simulink model "FocHFIGenerator"  (R2024a)
settings: Solver=FixedStepDiscrete  StartTime=0.0  StopTime=1  FixedStep=0.00005  RelTol=1e-3
values from neighbouring files (symbols this model uses):
  Max_Current = 10    [FocHFIGenerator.mat]    (also in NLFO_CodeGenerator.mat)
  Pole = 10    [FocHFIGenerator.mat]    (also in NLFO_CodeGenerator.mat = 7)
  UdInjectVal = 2.5    [FocHFIGenerator.mat]
undefined symbols (not defined in the file or in its folder): DiscIntNeverNeededParam
libraries: slpidlib x4
settings Model: Creator=张先生  LastModifiedBy=张先生
settings OptimizationCC: DefaultParameterBehavior=Inlined  UseDivisionForNetSlopeComputation=on  GainParamInheritBuiltInType=on  UseFloatMulNetSlope=on  InlineInvariantSignals=on  PassReuseOutputArgsAs=Individual arguments  ZeroExternalMemoryAtStartup=off  ZeroInternalMemoryAtStartup=off  NoFixptDivByZeroProtection=on  EfficientFloat2IntCast=on  LifeSpan=1  OptimizeBlockOrder=speed  DifferentSizesBufferReuse=on  EfficientTunableParamExpr=on
settings DebuggingCC: ParameterTunabilityLossMsg=error
settings HardwareCC: ProdBitPerPointer=32  ProdBitPerSizeT=32  ProdBitPerPtrDiffT=32  ProdLargestAtomicInteger=Long  ProdLargestAtomicFloat=Double  ProdWordSize=32  ProdLongLongMode=on  ProdHWDeviceType=ARM Compatible->ARM Cortex-M
settings SFSimCC: MATLABDynamicMemAlloc=off
settings RTWCC: Description=Embedded Coder  SystemTargetFile=ert.tlc  TemplateMakefile=ert_default_tmf  GenerateReport=on  LaunchReport=on
settings CodeAppCC: ForceParamTrailComments=on  IgnoreCustomStorageClasses=off  OperatorAnnotations=on  SimulinkDataObjDesc=on  SFDataObjDesc=on  CustomSymbolStrGlobalVar=rt$N$M  CustomSymbolStrType=$N$M  CustomSymbolStrFcn=$N$M$F  CustomSymbolStrMacro=$N$M  InsertBlockDesc=on
settings ERTTargetCC: TargetLangStandard=C99 (ISO)  CodeReplacementLibrary=ARM Cortex-M  GenerateSampleERTMain=on  IncludeMdlTerminateFcn=off  CombineSignalStateStructs=on  SupportComplex=off  SupportContinuousTime=on  InlinedParameterPlacement=NonHierarchical  ERTCustomFileTemplate=example_file_process.tlc  ERTFilePackagingFormat=CompactWithDataFile

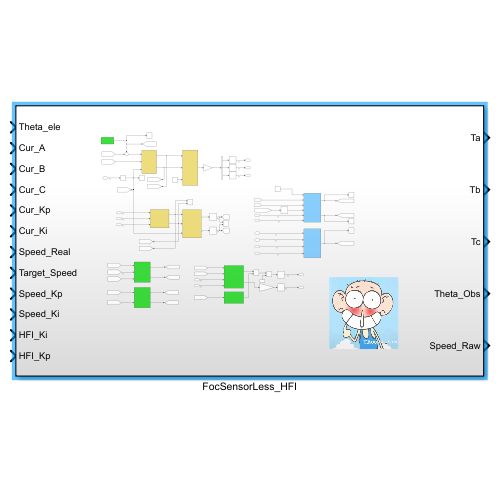
[thumbnail: Simulink's stored preview of the top-level diagram]
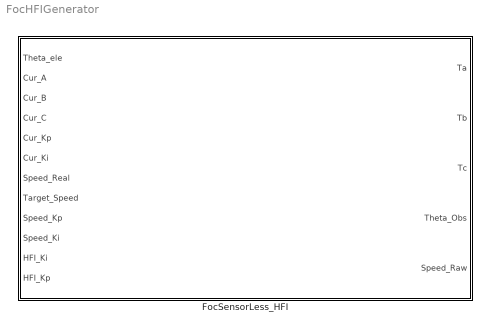
== system FocHFIGenerator ==
  FocSensorLess_HFI : Subsystem

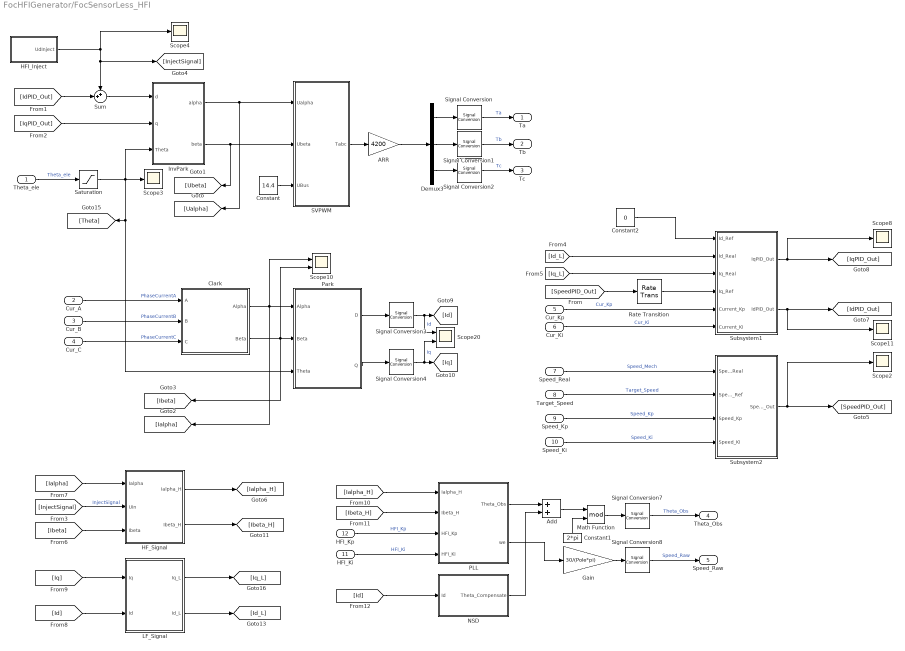
== system FocHFIGenerator/FocSensorLess_HFI ==
  Theta_ele : Inport
  Cur_A : Inport  Port=2
  Cur_B : Inport  Port=3
  Cur_C : Inport  Port=4
  Cur_Kp : Inport  Port=5
  Cur_Ki : Inport  Port=6
  Speed_Real : Inport  Port=7
  Target_Speed : Inport  Port=8
  Speed_Kp : Inport  Port=9
  Speed_Ki : Inport  Port=10
  HFI_Ki : Inport  Port=11
  HFI_Kp : Inport  Port=12
  ARR : Gain  Gain=4200
  Add : Sum
  Clark : Subsystem  TreatAsAtomicUnit=on
      settings: RTWSystemCode=Inline  RTWFcnNameOpts=Use subsystem name
      mask Display:
      | port_label('input',1,'a','texmode','on');
      | port_label('input',2,'b','texmode','on');
      | port_label('input',3,'c','texmode','on');
      | 
      | port_label('output',1,'\alpha','texmode','on');
      | port_label('output',2,'\beta','texmode','on');
      | 
      | fprintf('Clark');
  Constant : Constant  Value=14.4  OutDataTypeStr=single
  Constant1 : Constant  Value=2*pi  OutDataTypeStr=single
  Constant2 : Constant  Value=0  OutDataTypeStr=single
  Demux3 : Demux  Outputs=3
  Gain : Gain  Gain=30/(Pole*pi)
  HFI_Inject : Subsystem
  HF_Signal : Subsystem
  InvPark : Subsystem  TreatAsAtomicUnit=on
      settings: RTWFcnNameOpts=Use subsystem name
      mask Display:
      | port_label('input',1,'d','texmode','on');
      | port_label('input',2,'q','texmode','on');
      | port_label('input',3,'\theta','texmode','on');
      | 
      | port_label('output',1,'\alpha','texmode','on');
      | port_label('output',2,'\beta','texmode','on');
      | 
      | fprintf('Inverse\nPark')
  LF_Signal : Subsystem
  Math Function : Math  Operator=mod
  NSD : Subsystem
  PLL : Subsystem
  Park : Subsystem  TreatAsAtomicUnit=on
      settings: RTWFcnNameOpts=Use subsystem name
      mask Display:
      | port_label('input',1,'\alpha','texmode','on');
      | port_label('input',2, '\beta','texmode','on');
      | port_label('input',3, '\theta','texmode','on');
      | 
      | port_label('output',1,'d','texmode','on');
      | port_label('output',2,'q','texmode','on');
      | fprintf('Park');
  Rate Transition : RateTransition
  SVPWM : Subsystem  TreatAsAtomicUnit=on
  Saturation : Saturate  UpperLimit=2*pi-0.001  LowerLimit=-2*pi + 0.001
  Scope10 : Scope  NumInputPorts=2
  Scope{2..4,8,11} (5 alike) : Scope
  Scope20 : Scope  NumInputPorts=2
  Signal Conversion{,1..4,7..8} (7 alike) : SignalConversion  OverrideOpt=off
  Subsystem1 : Subsystem
  Subsystem2 : Subsystem
  Sum : Sum  Inputs=++|
  Ta : Outport
  Tb : Outport  Port=2
  Tc : Outport  Port=3
  Theta_Obs : Outport  Port=4
  Speed_Raw : Outport  Port=5
  wires:
  [Id_L] -> Subsystem1/2(Id_Real)
  InvPark/1(alpha) -> SVPWM/1(Ualpha), [Ualpha]
  InvPark/2(beta) -> SVPWM/2(Ubeta), [Ubeta]
  Saturation/1 -> [Theta], Park/3(Theta), Scope3/1, InvPark/3(Theta)
  Cur_Kp/1 -> Subsystem1/5(Current_Kp)  "Cur_Kp"
  SVPWM/1(Tabc) -> ARR/1
  Subsystem1/1(IqPID_Out) -> Scope8/1, [IqPID_Out]
  Theta_ele/1 -> Saturation/1  "Theta_ele"
  ARR/1 -> Demux3/1
  Cur_C/1 -> Clark/3(C)  "PhaseCurrentC"
  Park/1(D) -> Signal Conversion3/1
  Signal Conversion4/1 -> Scope20/2, [Iq]  "Iq"
  Cur_B/1 -> Clark/2(B)  "PhaseCurrentB"
  Signal Conversion2/1 -> Tc/1  "Tc"
  Signal Conversion3/1 -> Scope20/1, [Id]  "Id"
  Signal Conversion/1 -> Ta/1  "Ta"
  Cur_A/1 -> Clark/1(A)  "PhaseCurrentA"
  Demux3/2 -> Signal Conversion1/1
  Demux3/1 -> Signal Conversion/1
  Park/2(Q) -> Signal Conversion4/1
  [Iq_L] -> Subsystem1/3(Iq_Real)
  Demux3/3 -> Signal Conversion2/1
  Subsystem1/2(IdPID_Out) -> Scope11/1, [IdPID_Out]
  Signal Conversion1/1 -> Tb/1  "Tb"
  Constant/1 -> SVPWM/3(UBus)
  Cur_Ki/1 -> Subsystem1/6(Current_Ki)  "Cur_Ki"
  Subsystem2/1(SpeedPID_Out) -> Scope2/1, [SpeedPID_Out]
  [SpeedPID_Out] -> Rate Transition/1
  Speed_Real/1 -> Subsystem2/1(Speed_Real)  "Speed_Mech"
  Target_Speed/1 -> Subsystem2/2(Speed_Ref)  "Target_Speed"
  Speed_Kp/1 -> Subsystem2/3(Speed_Kp)  "Speed_Kp"
  Speed_Ki/1 -> Subsystem2/4(Speed_Ki)  "Speed_Ki"
  Rate Transition/1 -> Subsystem1/4(Iq_Ref)
  Clark/2(Beta) -> [Ibeta], Park/2(Beta), Scope10/2
  Clark/1(Alpha) -> [Ialpha], Park/1(Alpha), Scope10/1
  Sum/1 -> InvPark/1(d)
  HFI_Inject/1(UdInject) -> Scope4/1, Sum/1, [InjectSignal]
  HFI_Ki/1 -> PLL/4(HFI_Ki)  "HFI_Ki"
  HFI_Kp/1 -> PLL/3(HFI_Kp)  "HFI_Kp"
  [Ibeta_H] -> PLL/2(Ibeta_H)
  [Ialpha_H] -> PLL/1(Ialpha_H)
  PLL/1(Theta_Obs) -> Add/1
  NSD/1(Theta_Compensate) -> Add/2
  Constant1/1 -> Math Function/2
  Add/1 -> Math Function/1
  Math Function/1 -> Signal Conversion7/1
  PLL/2(we) -> Gain/1
  Signal Conversion7/1 -> Theta_Obs/1  "Theta_Obs"
  Signal Conversion8/1 -> Speed_Raw/1  "Speed_Raw"
  [Ibeta] -> HF_Signal/3(Ibeta)
  [Ialpha] -> HF_Signal/1(Ialpha)
  [InjectSignal] -> HF_Signal/2(Uin)  "InjectSignal"
  HF_Signal/2(Ibeta_H) -> [Ibeta_H]
  HF_Signal/1(Ialpha_H) -> [Ialpha_H]
  [Iq] -> LF_Signal/1(Iq)
  [Id] -> LF_Signal/2(Id)
  LF_Signal/1(Iq_L) -> [Iq_L]
  LF_Signal/2(Id_L) -> [Id_L]
  [Id] -> NSD/1(Id)
  Gain/1 -> Signal Conversion8/1
  Constant2/1 -> Subsystem1/1(Id_Ref)
  [IdPID_Out] -> Sum/2
  [IqPID_Out] -> InvPark/2(q)

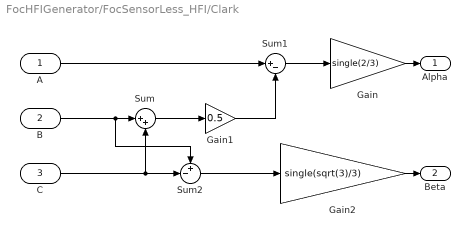
== system FocHFIGenerator/FocSensorLess_HFI/Clark ==
  A : Inport  OutDataTypeStr=single
  B : Inport  Port=2  OutDataTypeStr=single
  C : Inport  Port=3  OutDataTypeStr=single
  Gain : Gain  Gain=single(2/3)  OutDataTypeStr=single
  Gain1 : Gain  Gain=0.5  OutDataTypeStr=single
  Gain2 : Gain  Gain=single(sqrt(3)/3)  OutDataTypeStr=single
  Sum : Sum  Inputs=|++  OutDataTypeStr=single
  Sum1 : Sum  Inputs=|+-  OutDataTypeStr=single
  Sum2 : Sum  Inputs=+-|  OutDataTypeStr=single
  Alpha : Outport  OutDataTypeStr=single
  Beta : Outport  Port=2  OutDataTypeStr=single
  wires:
  Sum/1 -> Gain1/1
  Gain2/1 -> Beta/1
  B/1 -> Sum2/1, Sum/1
  Gain1/1 -> Sum1/2
  Gain/1 -> Alpha/1
  Sum2/1 -> Gain2/1
  C/1 -> Sum2/2, Sum/2
  A/1 -> Sum1/1
  Sum1/1 -> Gain/1

== system FocHFIGenerator/FocSensorLess_HFI/HFI_Inject ==
  note: 前0.2S进行极性辨识
  Scope : Scope
  Scope1 : Scope  NumInputPorts=2
  Subsystem : Subsystem
  Subsystem4 : Subsystem
  Sum1 : Sum  Inputs=++|
  UdInject : Outport
  wires:
  Subsystem/1(Ud_Inject) -> Scope1/2, Sum1/2
  Subsystem4/1(NDS_Signal) -> Scope1/1, Sum1/1
  Sum1/1 -> Scope/1, UdInject/1

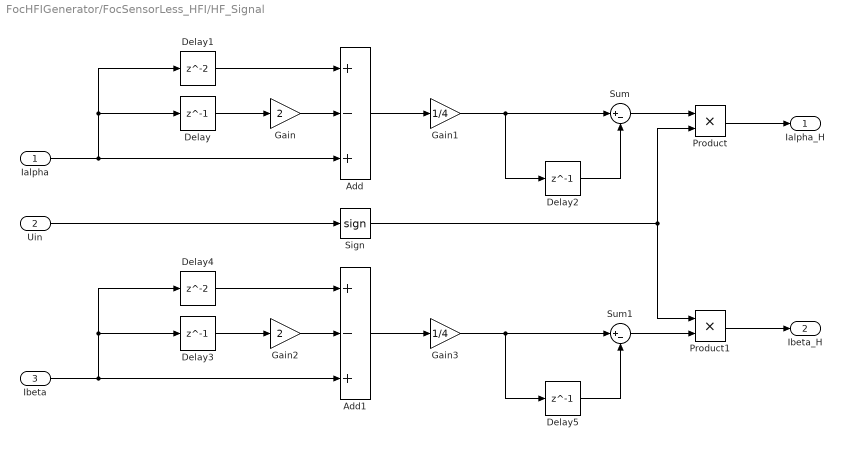
== system FocHFIGenerator/FocSensorLess_HFI/HF_Signal ==
  Ialpha : Inport
  Uin : Inport  Port=2
  Ibeta : Inport  Port=3
  Add : Sum  Inputs=+-+
  Add1 : Sum  Inputs=+-+
  Delay{,2..3,5} (4 alike) : Delay  DelayLength=1
  Delay1 : Delay
  Delay4 : Delay
  Gain : Gain  Gain=2
  Gain1 : Gain  Gain=1/4
  Gain2 : Gain  Gain=2
  Gain3 : Gain  Gain=1/4
  Product : Product
  Product1 : Product
  Sign : Signum
  Sum : Sum  Inputs=|+-
  Sum1 : Sum  Inputs=|+-
  Ialpha_H : Outport
  Ibeta_H : Outport  Port=2
  wires:
  Delay/1 -> Gain/1
  Delay1/1 -> Add/1
  Gain/1 -> Add/2
  Ialpha/1 -> Add/3, Delay1/1, Delay/1
  Add/1 -> Gain1/1
  Gain1/1 -> Delay2/1, Sum/1
  Delay2/1 -> Sum/2
  Sum/1 -> Product/1
  Product/1 -> Ialpha_H/1
  Uin/1 -> Sign/1
  Sign/1 -> Product1/1, Product/2
  Product1/1 -> Ibeta_H/1
  Add1/1 -> Gain3/1
  Delay5/1 -> Sum1/2
  Gain3/1 -> Delay5/1, Sum1/1
  Delay4/1 -> Add1/1
  Gain2/1 -> Add1/2
  Ibeta/1 -> Add1/3, Delay4/1, Delay3/1
  Delay3/1 -> Gain2/1
  Sum1/1 -> Product1/2

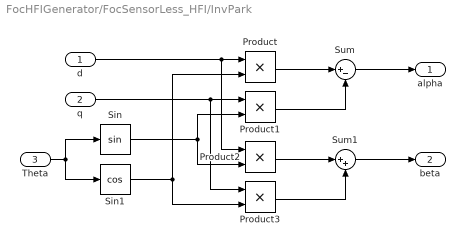
== system FocHFIGenerator/FocSensorLess_HFI/InvPark ==
  d : Inport  OutDataTypeStr=single
  q : Inport  Port=2  OutDataTypeStr=single
  Theta : Inport  Port=3  OutDataTypeStr=single
  Product{,1..3} (4 alike) : Product  OutDataTypeStr=single
  Sin : Trigonometry  ApproximationMethod=Lookup  TableDataTypeStr=single
  Sin1 : Trigonometry  Operator=cos  ApproximationMethod=Lookup  TableDataTypeStr=single
  Sum : Sum  Inputs=|+-  OutDataTypeStr=single
  Sum1 : Sum  Inputs=|++  OutDataTypeStr=single
  alpha : Outport  OutDataTypeStr=single
  beta : Outport  Port=2  OutDataTypeStr=single
  wires:
  Sum/1 -> alpha/1
  Theta/1 -> Sin1/1, Sin/1
  d/1 -> Product2/1, Product/1
  Sin1/1 -> Product/2, Product3/2
  q/1 -> Product3/1, Product1/1
  Sin/1 -> Product1/2, Product2/2
  Product/1 -> Sum/1
  Product1/1 -> Sum/2
  Product2/1 -> Sum1/1
  Product3/1 -> Sum1/2
  Sum1/1 -> beta/1

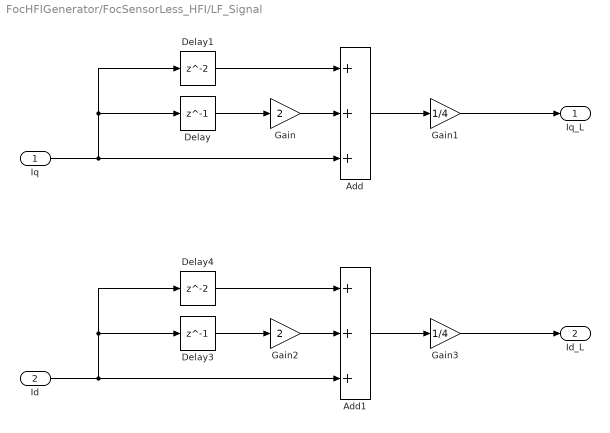
== system FocHFIGenerator/FocSensorLess_HFI/LF_Signal ==
  Iq : Inport
  Id : Inport  Port=2
  Add : Sum  Inputs=+++
  Add1 : Sum  Inputs=+++
  Delay : Delay  DelayLength=1
  Delay1 : Delay
  Delay3 : Delay  DelayLength=1
  Delay4 : Delay
  Gain : Gain  Gain=2
  Gain1 : Gain  Gain=1/4
  Gain2 : Gain  Gain=2
  Gain3 : Gain  Gain=1/4
  Iq_L : Outport
  Id_L : Outport  Port=2
  wires:
  Delay/1 -> Gain/1
  Delay1/1 -> Add/1
  Gain/1 -> Add/2
  Iq/1 -> Add/3, Delay1/1, Delay/1
  Add/1 -> Gain1/1
  Gain1/1 -> Iq_L/1
  Gain3/1 -> Id_L/1
  Add1/1 -> Gain3/1
  Delay4/1 -> Add1/1
  Gain2/1 -> Add1/2
  Id/1 -> Add1/3, Delay4/1, Delay3/1
  Delay3/1 -> Gain2/1

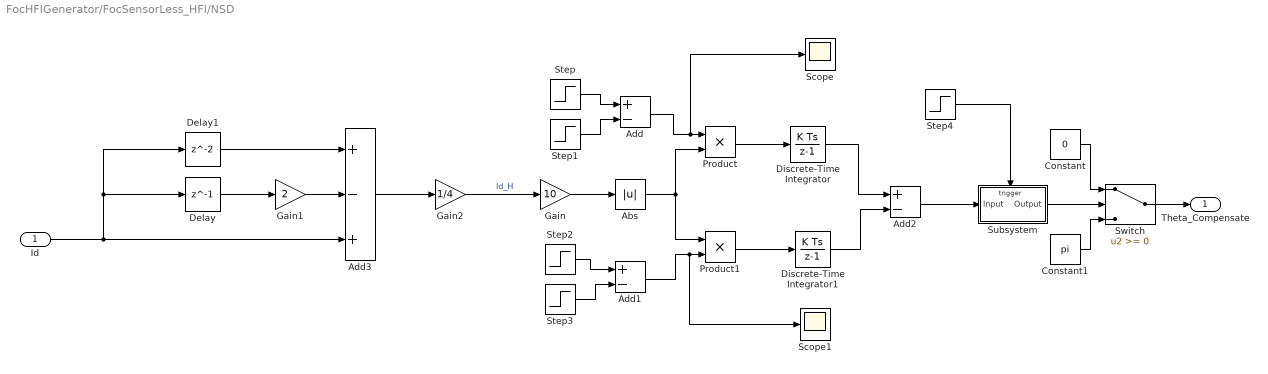
== system FocHFIGenerator/FocSensorLess_HFI/NSD ==
  Id : Inport
  Abs : Abs  OutDataTypeStr=single  SaturateOnIntegerOverflow=off
  Add : Sum  Inputs=+-  OutDataTypeStr=single  AccumDataTypeStr=single
  Add1 : Sum  Inputs=+-  OutDataTypeStr=single  AccumDataTypeStr=single
  Add2 : Sum  Inputs=+-  OutDataTypeStr=single  AccumDataTypeStr=single
  Add3 : Sum  Inputs=+-+
  Constant : Constant  Value=0  OutDataTypeStr=single
  Constant1 : Constant  Value=pi  OutDataTypeStr=single
  Delay : Delay  DelayLength=1
  Delay1 : Delay
  Discrete-Time Integrator : DiscreteIntegrator  SampleTime=-1  OutDataTypeStr=single  ICPrevOutput=DiscIntNeverNeededParam  ICPrevScaledInput=DiscIntNeverNeededParam
  Discrete-Time Integrator1 : DiscreteIntegrator  SampleTime=-1  OutDataTypeStr=single  ICPrevOutput=DiscIntNeverNeededParam  ICPrevScaledInput=DiscIntNeverNeededParam
  Gain : Gain  Gain=10
  Gain1 : Gain  Gain=2
  Gain2 : Gain  Gain=1/4
  Product : Product  OutDataTypeStr=single
  Product1 : Product  OutDataTypeStr=single
  Scope : Scope
  Scope1 : Scope
  Step : Step  Time=0.1  OutDataTypeStr=single  SampleTime=0
  Step1 : Step  Time=0.11  OutDataTypeStr=single  SampleTime=0
  Step2 : Step  Time=0.13  After=-1  OutDataTypeStr=single  SampleTime=0
  Step3 : Step  Time=0.14  After=-1  OutDataTypeStr=single  SampleTime=0
  Step4 : Step  Time=0.15  SampleTime=0
  Subsystem : Subsystem
  Switch : Switch  OutDataTypeStr=single  SaturateOnIntegerOverflow=off  InputSameDT=off
  Theta_Compensate : Outport
  wires:
  Gain/1 -> Abs/1
  Step/1 -> Add/1
  Step1/1 -> Add/2
  Step2/1 -> Add1/1
  Step3/1 -> Add1/2
  Add/1 -> Scope/1, Product/1
  Add1/1 -> Scope1/1, Product1/2
  Abs/1 -> Product1/1, Product/2
  Product/1 -> Discrete-Time Integrator/1
  Product1/1 -> Discrete-Time Integrator1/1
  Discrete-Time Integrator/1 -> Add2/1
  Discrete-Time Integrator1/1 -> Add2/2
  Step4/1 -> Subsystem/Trigger
  Add2/1 -> Subsystem/1(Input)
  Subsystem/1(Output) -> Switch/2
  Constant/1 -> Switch/1
  Constant1/1 -> Switch/3
  Switch/1 -> Theta_Compensate/1
  Id/1 -> Add3/3, Delay1/1, Delay/1
  Gain1/1 -> Add3/2
  Delay1/1 -> Add3/1
  Add3/1 -> Gain2/1
  Delay/1 -> Gain1/1
  Gain2/1 -> Gain/1  "Id_H"

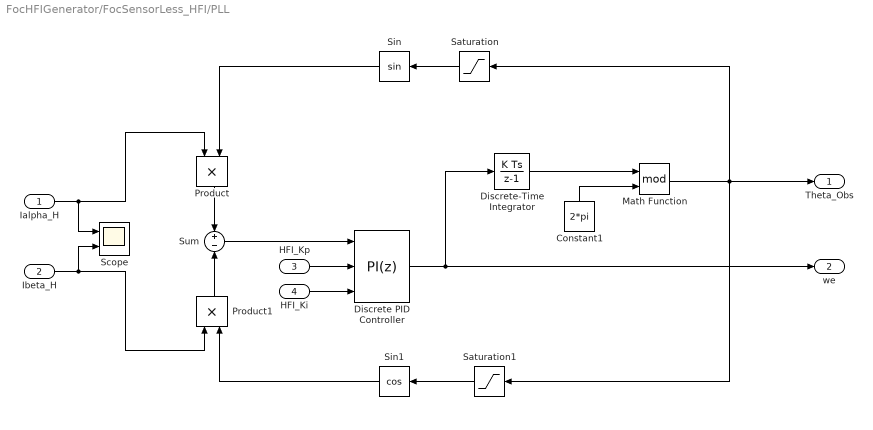
== system FocHFIGenerator/FocSensorLess_HFI/PLL ==
  Ialpha_H : Inport
  Ibeta_H : Inport  Port=2
  HFI_Kp : Inport  Port=3
  HFI_Ki : Inport  Port=4
  Constant1 : Constant  Value=2*pi  OutDataTypeStr=single
  Discrete PID Controller : slpidlib/PID Controller  Controller=PI  Form=Parallel  TimeDomain=Discrete-time  UseExternalTs=off  SampleTime=-1  IntegratorMethod=Forward Euler  FilterMethod=Forward Euler  ControllerParametersSource=external  P=10  I=1000  UseKiTs=off  D=0  UseExternalDerivativeSource=off  N=100  UseFilter=on  TunerSelectOption=Transfer Function Based (PID Tuner App)  InitialConditionSource=internal  InitialConditionForIntegrator=0  InitialConditionForFilter=0  DifferentiatorICPrevScaledInput=0  ExternalReset=none  TrackingMode=off  Kt=1  LimitOutput=off  SatLimitsSource=internal  UpperSaturationLimit=pi*2  LowerSaturationLimit=-pi*2  LinearizeAsGain=on  AntiWindupMode=clamping  Kb=1  LimitIntegrator=off  UpperIntegratorSaturationLimit=inf  LowerIntegratorSaturationLimit=-inf  PGainOutDataTypeStr=single  PProdOutDataTypeStr=single  POutMin=[]  POutMax=[]  IGainOutDataTypeStr=single  IProdOutDataTypeStr=single  IOutMin=[]  IOutMax=[]  DOutMin=[]  DOutMax=[]  NOutMin=[]  NOutMax=[]  SumOutDataTypeStr=single  SumOutMin=[]  SumOutMax=[]  SaturationOutMin=[]  SaturationOutMax=[]  PParamMin=[]  PParamMax=[]  IParamMin=[]  IParamMax=[]  DParamMin=[]  DParamMax=[]  NParamMin=[]  NParamMax=[]  KbParamMin=[]  KbParamMax=[]  KtParamMin=[]  KtParamMax=[]  KbOutMin=[]  KbOutMax=[]  KtOutMin=[]  KtOutMax=[]  IntegratorOutMin=[]  IntegratorOutMax=[]  FilterOutMin=[]  FilterOutMax=[]  SumI1OutMin=[]  SumI1OutMax=[]  SumI2OutMin=[]  SumI2OutMax=[]  SumI3OutMin=[]  SumI3OutMax=[]  SumI4OutMin=[]  SumI4OutMax=[]  SumDOutMin=[]  SumDOutMax=[]  DifferentiatorOutMin=[]  DifferentiatorOutMax=[]  FilterDiffOutCoefMin=[]  FilterDiffOutCoefMax=[]  ReciprocalOutMin=[]  ReciprocalOutMax=[]  SumDenOutMin=[]  SumDenOutMax=[]  SumNumOutMin=[]  SumNumOutMax=[]  DivideOutMin=[]  DivideOutMax=[]  UdiffTsProdOutMin=[]  UdiffTsProdOutMax=[]  NTsProdOutMin=[]  NTsProdOutMax=[]  UintegralTsProdOutMin=[]  UintegralTsProdOutMax=[]  UngainTsProdOutMin=[]  UngainTsProdOutMax=[]  ClampingZeroOutDataTypeStr=Inherit: Inherit via back propagation  ClampingZeroOutMin=[]  ClampingZeroOutMax=[]  FilterDenConstantOutDataTypeStr=Inherit: Inherit via back propagation  FilterDenConstantOutMin=[]  FilterDenConstantOutMax=[]  PCopyOutDataTypeStr=Inherit: Inherit via back propagation  PCopyOutMin=[]  PCopyOutMax=[]  NCopyOutDataTypeStr=Inherit: Inherit via back propagation  NCopyOutMin=[]  NCopyOutMax=[]  IntegratorContinuousStateAttributes=''  IntegratorStateMustResolveToSignalObject=off  IntegratorRTWStateStorageClass=Auto  FilterContinuousStateAttributes=''  FilterStateMustResolveToSignalObject=off  FilterRTWStateStorageClass=Auto  ParallelPVariant=ExternalParameters  IdealPVariant=Disabled  IVariant=ExternalParameters  DVariant=Disabled  IntegratorVariant=Discrete  SatVariant=Disabled  AWVariant=Passthrough  PCopyVariant=Disabled  TRVariant=Disabled  FdbkBlocksVariant=Forward  IdealPFdbkVariant=Disabled  SatFdbkVariant=Disabled  DerivativeFilterVariant=Disabled  NVariant=Disabled  NCopyVariant=Disabled_SignalSpec  FilterICVariant=Disabled  IntegratorICVariant=InternalICs  ExternalResetVariant=Disabled  TRSumVariant=Passthrough  SumFdbkVariant=Disabled  SumVariant=Sum_PI  TsampFilterVariant=InternalTs  TsampNgainVariant=Passthrough  TsampIntegralVariant=Disabled_SignalSpec  ExternalSaturationOutDataTypeStr=Inherit: Same as second input  DerivativeSourceVariant=Disabled
      settings: LibrarySourceBlock=simulink/Discrete/Discrete PID Controller
  Discrete-Time Integrator : DiscreteIntegrator  SampleTime=-1  OutDataTypeStr=single  ICPrevOutput=DiscIntNeverNeededParam  ICPrevScaledInput=DiscIntNeverNeededParam
  Math Function : Math  Operator=mod
  Product : Product
  Product1 : Product
  Saturation : Saturate  UpperLimit=2*pi - 0.001  LowerLimit=-2*pi + 0.001  OutDataTypeStr=single
  Saturation1 : Saturate  UpperLimit=2*pi - 0.001  LowerLimit=-2*pi + 0.001  OutDataTypeStr=single
  Scope : Scope  NumInputPorts=2
  Sin : Trigonometry  ApproximationMethod=Lookup
  Sin1 : Trigonometry  Operator=cos  ApproximationMethod=Lookup
  Sum : Sum  Inputs=+|-
  Theta_Obs : Outport
  we : Outport  Port=2
  wires:
  Product/1 -> Sum/1
  Product1/1 -> Sum/2
  Ialpha_H/1 -> Product/1, Scope/1
  Ibeta_H/1 -> Scope/2, Product1/1
  Sum/1 -> Discrete PID Controller/1
  Discrete PID Controller/1 -> Discrete-Time Integrator/1, we/1
  Discrete-Time Integrator/1 -> Math Function/1
  Sin/1 -> Product/2
  Sin1/1 -> Product1/2
  Saturation/1 -> Sin/1
  Saturation1/1 -> Sin1/1
  Constant1/1 -> Math Function/2
  Math Function/1 -> Theta_Obs/1, Saturation/1, Saturation1/1
  HFI_Kp/1 -> Discrete PID Controller/2
  HFI_Ki/1 -> Discrete PID Controller/3

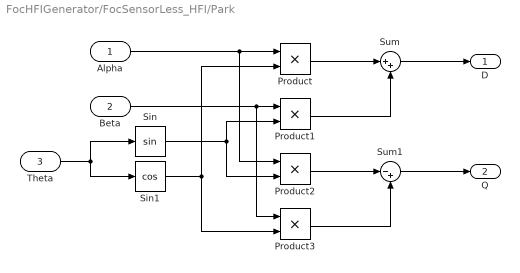
== system FocHFIGenerator/FocSensorLess_HFI/Park ==
  Alpha : Inport  OutDataTypeStr=single
  Beta : Inport  Port=2  OutDataTypeStr=single
  Theta : Inport  Port=3  OutDataTypeStr=single
  Product{,1..3} (4 alike) : Product  OutDataTypeStr=single
  Sin : Trigonometry  ApproximationMethod=Lookup  TableDataTypeStr=single
  Sin1 : Trigonometry  Operator=cos  ApproximationMethod=Lookup  TableDataTypeStr=single
  Sum : Sum  Inputs=|++  OutDataTypeStr=single
  Sum1 : Sum  Inputs=|-+  OutDataTypeStr=single
  D : Outport  OutDataTypeStr=single
  Q : Outport  Port=2  OutDataTypeStr=single
  wires:
  Beta/1 -> Product3/1, Product1/1
  Alpha/1 -> Product2/1, Product/1
  Theta/1 -> Sin1/1, Sin/1
  Sin1/1 -> Product/2, Product3/2
  Sin/1 -> Product1/2, Product2/2
  Product/1 -> Sum/1
  Product1/1 -> Sum/2
  Sum/1 -> D/1
  Product2/1 -> Sum1/1
  Product3/1 -> Sum1/2
  Sum1/1 -> Q/1

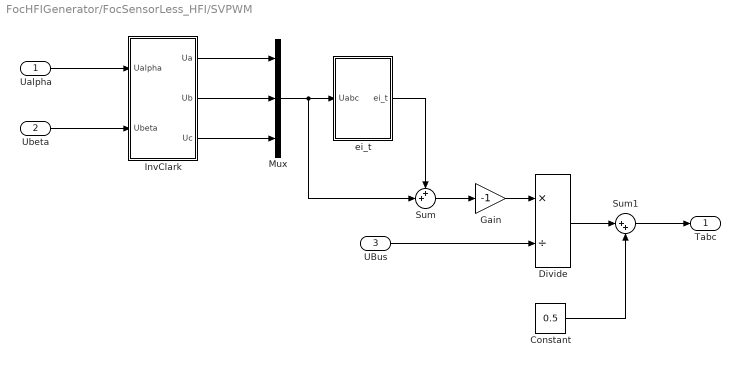
== system FocHFIGenerator/FocSensorLess_HFI/SVPWM ==
  Ualpha : Inport  OutDataTypeStr=single
  Ubeta : Inport  Port=2  OutDataTypeStr=single
  UBus : Inport  Port=3  OutDataTypeStr=single
  Constant : Constant  Value=0.5  OutDataTypeStr=single
  Divide : Product  Inputs=*/  OutDataTypeStr=single
  Gain : Gain  Gain=-1  OutDataTypeStr=single
  InvClark : Subsystem
  Mux : Mux  Inputs=3
  Sum : Sum  Inputs=++|  OutDataTypeStr=single
  Sum1 : Sum  Inputs=|++  OutDataTypeStr=single
  ei_t : Subsystem
  Tabc : Outport  OutDataTypeStr=single
  wires:
  Ualpha/1 -> InvClark/1(Ualpha)
  Ubeta/1 -> InvClark/2(Ubeta)
  ei_t/1(ei_t) -> Sum/1
  InvClark/1(Ua) -> Mux/1
  InvClark/2(Ub) -> Mux/2
  InvClark/3(Uc) -> Mux/3
  Sum/1 -> Gain/1
  Mux/1 -> Sum/2, ei_t/1(Uabc)
  Divide/1 -> Sum1/1
  Constant/1 -> Sum1/2
  UBus/1 -> Divide/2
  Gain/1 -> Divide/1
  Sum1/1 -> Tabc/1

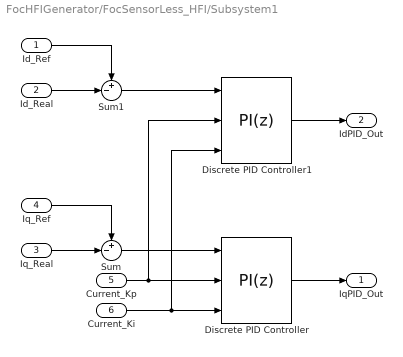
== system FocHFIGenerator/FocSensorLess_HFI/Subsystem1 ==
  Id_Ref : Inport
  Id_Real : Inport  Port=2
  Iq_Real : Inport  Port=3
  Iq_Ref : Inport  Port=4
  Current_Kp : Inport  Port=5
  Current_Ki : Inport  Port=6
  Discrete PID Controller : slpidlib/PID Controller  Controller=PI  Form=Parallel  TimeDomain=Discrete-time  UseExternalTs=off  SampleTime=-1  IntegratorMethod=Forward Euler  FilterMethod=Forward Euler  ControllerParametersSource=external  P=1  I=1  UseKiTs=off  D=0  UseExternalDerivativeSource=off  N=100  UseFilter=on  TunerSelectOption=Transfer Function Based (PID Tuner App)  InitialConditionSource=internal  InitialConditionForIntegrator=0  InitialConditionForFilter=0  DifferentiatorICPrevScaledInput=0  ExternalReset=none  TrackingMode=off  Kt=1  LimitOutput=on  SatLimitsSource=internal  UpperSaturationLimit=6  LowerSaturationLimit=-6  LinearizeAsGain=off  AntiWindupMode=clamping  Kb=1  LimitIntegrator=off  UpperIntegratorSaturationLimit=inf  LowerIntegratorSaturationLimit=-inf  SaturateOnIntegerOverflow=on  PGainOutDataTypeStr=single  PProdOutDataTypeStr=single  POutMin=[]  POutMax=[]  IGainOutDataTypeStr=single  IProdOutDataTypeStr=single  IOutMin=[]  IOutMax=[]  DOutMin=[]  DOutMax=[]  NOutMin=[]  NOutMax=[]  SumOutDataTypeStr=single  SumOutMin=[]  SumOutMax=[]  SaturationOutMin=[]  SaturationOutMax=[]  PParamMin=[]  PParamMax=[]  IParamMin=[]  IParamMax=[]  DParamMin=[]  DParamMax=[]  NParamMin=[]  NParamMax=[]  KbParamMin=[]  KbParamMax=[]  KtParamMin=[]  KtParamMax=[]  KbOutMin=[]  KbOutMax=[]  KtOutMin=[]  KtOutMax=[]  IntegratorOutMin=[]  IntegratorOutMax=[]  FilterOutMin=[]  FilterOutMax=[]  SumI1OutMin=[]  SumI1OutMax=[]  SumI2OutMin=[]  SumI2OutMax=[]  SumI3OutMin=[]  SumI3OutMax=[]  SumI4OutMin=[]  SumI4OutMax=[]  SumDOutMin=[]  SumDOutMax=[]  DifferentiatorOutMin=[]  DifferentiatorOutMax=[]  FilterDiffOutCoefMin=[]  FilterDiffOutCoefMax=[]  ReciprocalOutMin=[]  ReciprocalOutMax=[]  SumDenOutMin=[]  SumDenOutMax=[]  SumNumOutMin=[]  SumNumOutMax=[]  DivideOutMin=[]  DivideOutMax=[]  UdiffTsProdOutMin=[]  UdiffTsProdOutMax=[]  NTsProdOutMin=[]  NTsProdOutMax=[]  UintegralTsProdOutMin=[]  UintegralTsProdOutMax=[]  UngainTsProdOutMin=[]  UngainTsProdOutMax=[]  ClampingZeroOutDataTypeStr=Inherit: Inherit via back propagation  ClampingZeroOutMin=[]  ClampingZeroOutMax=[]  FilterDenConstantOutDataTypeStr=Inherit: Inherit via back propagation  FilterDenConstantOutMin=[]  FilterDenConstantOutMax=[]  PCopyOutDataTypeStr=Inherit: Inherit via back propagation  PCopyOutMin=[]  PCopyOutMax=[]  NCopyOutDataTypeStr=Inherit: Inherit via back propagation  NCopyOutMin=[]  NCopyOutMax=[]  IntegratorContinuousStateAttributes=''  IntegratorStateMustResolveToSignalObject=off  IntegratorRTWStateStorageClass=Auto  FilterContinuousStateAttributes=''  FilterStateMustResolveToSignalObject=off  FilterRTWStateStorageClass=Auto  ParallelPVariant=ExternalParameters  IdealPVariant=Disabled  IVariant=ExternalParameters  DVariant=Disabled  IntegratorVariant=Discrete  SatVariant=Enabled  AWVariant=DiscClampingParallel  PCopyVariant=Disabled  TRVariant=Disabled  FdbkBlocksVariant=Forward  IdealPFdbkVariant=Disabled  SatFdbkVariant=Disabled  DerivativeFilterVariant=Disabled  NVariant=Disabled  NCopyVariant=Disabled_SignalSpec  FilterICVariant=Disabled  IntegratorICVariant=InternalICs  ExternalResetVariant=Disabled  TRSumVariant=Passthrough  SumFdbkVariant=Disabled  SumVariant=Sum_PI  TsampFilterVariant=InternalTs  TsampNgainVariant=Passthrough  TsampIntegralVariant=Disabled_SignalSpec  ExternalSaturationOutDataTypeStr=Inherit: Same as second input  DerivativeSourceVariant=Disabled
      settings: LibrarySourceBlock=simulink/Discrete/Discrete PID Controller
  Discrete PID Controller1 : slpidlib/PID Controller  Controller=PI  Form=Parallel  TimeDomain=Discrete-time  UseExternalTs=off  SampleTime=-1  IntegratorMethod=Forward Euler  FilterMethod=Forward Euler  ControllerParametersSource=external  P=1  I=1  UseKiTs=off  D=0  UseExternalDerivativeSource=off  N=100  UseFilter=on  TunerSelectOption=Transfer Function Based (PID Tuner App)  InitialConditionSource=internal  InitialConditionForIntegrator=0  InitialConditionForFilter=0  DifferentiatorICPrevScaledInput=0  ExternalReset=none  TrackingMode=off  Kt=1  LimitOutput=on  SatLimitsSource=internal  UpperSaturationLimit=6  LowerSaturationLimit=-6  LinearizeAsGain=off  AntiWindupMode=clamping  Kb=1  LimitIntegrator=off  UpperIntegratorSaturationLimit=inf  LowerIntegratorSaturationLimit=-inf  SaturateOnIntegerOverflow=on  PGainOutDataTypeStr=single  PProdOutDataTypeStr=single  POutMin=[]  POutMax=[]  IGainOutDataTypeStr=single  IProdOutDataTypeStr=single  IOutMin=[]  IOutMax=[]  DOutMin=[]  DOutMax=[]  NOutMin=[]  NOutMax=[]  SumOutDataTypeStr=single  SumOutMin=[]  SumOutMax=[]  SaturationOutMin=[]  SaturationOutMax=[]  PParamMin=[]  PParamMax=[]  IParamMin=[]  IParamMax=[]  DParamMin=[]  DParamMax=[]  NParamMin=[]  NParamMax=[]  KbParamMin=[]  KbParamMax=[]  KtParamMin=[]  KtParamMax=[]  KbOutMin=[]  KbOutMax=[]  KtOutMin=[]  KtOutMax=[]  IntegratorOutMin=[]  IntegratorOutMax=[]  FilterOutMin=[]  FilterOutMax=[]  SumI1OutMin=[]  SumI1OutMax=[]  SumI2OutMin=[]  SumI2OutMax=[]  SumI3OutMin=[]  SumI3OutMax=[]  SumI4OutMin=[]  SumI4OutMax=[]  SumDOutMin=[]  SumDOutMax=[]  DifferentiatorOutMin=[]  DifferentiatorOutMax=[]  FilterDiffOutCoefMin=[]  FilterDiffOutCoefMax=[]  ReciprocalOutMin=[]  ReciprocalOutMax=[]  SumDenOutMin=[]  SumDenOutMax=[]  SumNumOutMin=[]  SumNumOutMax=[]  DivideOutMin=[]  DivideOutMax=[]  UdiffTsProdOutMin=[]  UdiffTsProdOutMax=[]  NTsProdOutMin=[]  NTsProdOutMax=[]  UintegralTsProdOutMin=[]  UintegralTsProdOutMax=[]  UngainTsProdOutMin=[]  UngainTsProdOutMax=[]  ClampingZeroOutDataTypeStr=Inherit: Inherit via back propagation  ClampingZeroOutMin=[]  ClampingZeroOutMax=[]  FilterDenConstantOutDataTypeStr=Inherit: Inherit via back propagation  FilterDenConstantOutMin=[]  FilterDenConstantOutMax=[]  PCopyOutDataTypeStr=Inherit: Inherit via back propagation  PCopyOutMin=[]  PCopyOutMax=[]  NCopyOutDataTypeStr=Inherit: Inherit via back propagation  NCopyOutMin=[]  NCopyOutMax=[]  IntegratorContinuousStateAttributes=''  IntegratorStateMustResolveToSignalObject=off  IntegratorRTWStateStorageClass=Auto  FilterContinuousStateAttributes=''  FilterStateMustResolveToSignalObject=off  FilterRTWStateStorageClass=Auto  ParallelPVariant=ExternalParameters  IdealPVariant=Disabled  IVariant=ExternalParameters  DVariant=Disabled  IntegratorVariant=Discrete  SatVariant=Enabled  AWVariant=DiscClampingParallel  PCopyVariant=Disabled  TRVariant=Disabled  FdbkBlocksVariant=Forward  IdealPFdbkVariant=Disabled  SatFdbkVariant=Disabled  DerivativeFilterVariant=Disabled  NVariant=Disabled  NCopyVariant=Disabled_SignalSpec  FilterICVariant=Disabled  IntegratorICVariant=InternalICs  ExternalResetVariant=Disabled  TRSumVariant=Passthrough  SumFdbkVariant=Disabled  SumVariant=Sum_PI  TsampFilterVariant=InternalTs  TsampNgainVariant=Passthrough  TsampIntegralVariant=Disabled_SignalSpec  ExternalSaturationOutDataTypeStr=Inherit: Same as second input  DerivativeSourceVariant=Disabled
      settings: LibrarySourceBlock=simulink/Discrete/Discrete PID Controller
  Sum : Sum  Inputs=+-|
  Sum1 : Sum  Inputs=+-|
  IqPID_Out : Outport
  IdPID_Out : Outport  Port=2
  wires:
  Sum/1 -> Discrete PID Controller/1
  Current_Kp/1 -> Discrete PID Controller/2, Discrete PID Controller1/2
  Iq_Ref/1 -> Sum/1
  Discrete PID Controller/1 -> IqPID_Out/1
  Current_Ki/1 -> Discrete PID Controller/3, Discrete PID Controller1/3
  Iq_Real/1 -> Sum/2
  Id_Ref/1 -> Sum1/1
  Id_Real/1 -> Sum1/2
  Sum1/1 -> Discrete PID Controller1/1
  Discrete PID Controller1/1 -> IdPID_Out/1

== system FocHFIGenerator/FocSensorLess_HFI/Subsystem2 ==
  Speed_Real : Inport
  Speed_Ref : Inport  Port=2
  Speed_Kp : Inport  Port=3
  Speed_Ki : Inport  Port=4
  Discrete PID Controller : slpidlib/PID Controller  Controller=PI  Form=Parallel  TimeDomain=Discrete-time  UseExternalTs=off  SampleTime=0.00025  IntegratorMethod=Forward Euler  FilterMethod=Forward Euler  ControllerParametersSource=external  P=1  I=1  UseKiTs=off  D=0  UseExternalDerivativeSource=off  N=100  UseFilter=on  TunerSelectOption=Transfer Function Based (PID Tuner App)  InitialConditionSource=internal  InitialConditionForIntegrator=0  InitialConditionForFilter=0  DifferentiatorICPrevScaledInput=0  ExternalReset=none  TrackingMode=off  Kt=1  LimitOutput=on  SatLimitsSource=internal  UpperSaturationLimit=Max_Current  LowerSaturationLimit=-Max_Current  LinearizeAsGain=off  AntiWindupMode=clamping  Kb=1  LimitIntegrator=off  UpperIntegratorSaturationLimit=inf  LowerIntegratorSaturationLimit=-inf  SaturateOnIntegerOverflow=on  PGainOutDataTypeStr=single  PProdOutDataTypeStr=single  POutMin=[]  POutMax=[]  IGainOutDataTypeStr=single  IProdOutDataTypeStr=single  IOutMin=[]  IOutMax=[]  DOutMin=[]  DOutMax=[]  NOutMin=[]  NOutMax=[]  SumOutDataTypeStr=single  SumOutMin=[]  SumOutMax=[]  SaturationOutMin=[]  SaturationOutMax=[]  PParamMin=[]  PParamMax=[]  IParamMin=[]  IParamMax=[]  DParamMin=[]  DParamMax=[]  NParamMin=[]  NParamMax=[]  KbParamMin=[]  KbParamMax=[]  KtParamMin=[]  KtParamMax=[]  KbOutMin=[]  KbOutMax=[]  KtOutMin=[]  KtOutMax=[]  IntegratorOutMin=[]  IntegratorOutMax=[]  FilterOutMin=[]  FilterOutMax=[]  SumI1OutMin=[]  SumI1OutMax=[]  SumI2OutMin=[]  SumI2OutMax=[]  SumI3OutMin=[]  SumI3OutMax=[]  SumI4OutMin=[]  SumI4OutMax=[]  SumDOutMin=[]  SumDOutMax=[]  DifferentiatorOutMin=[]  DifferentiatorOutMax=[]  FilterDiffOutCoefMin=[]  FilterDiffOutCoefMax=[]  ReciprocalOutMin=[]  ReciprocalOutMax=[]  SumDenOutMin=[]  SumDenOutMax=[]  SumNumOutMin=[]  SumNumOutMax=[]  DivideOutMin=[]  DivideOutMax=[]  UdiffTsProdOutMin=[]  UdiffTsProdOutMax=[]  NTsProdOutMin=[]  NTsProdOutMax=[]  UintegralTsProdOutMin=[]  UintegralTsProdOutMax=[]  UngainTsProdOutMin=[]  UngainTsProdOutMax=[]  ClampingZeroOutDataTypeStr=Inherit: Inherit via back propagation  ClampingZeroOutMin=[]  ClampingZeroOutMax=[]  FilterDenConstantOutDataTypeStr=Inherit: Inherit via back propagation  FilterDenConstantOutMin=[]  FilterDenConstantOutMax=[]  PCopyOutDataTypeStr=Inherit: Inherit via back propagation  PCopyOutMin=[]  PCopyOutMax=[]  NCopyOutDataTypeStr=Inherit: Inherit via back propagation  NCopyOutMin=[]  NCopyOutMax=[]  IntegratorContinuousStateAttributes=''  IntegratorStateMustResolveToSignalObject=off  IntegratorRTWStateStorageClass=Auto  FilterContinuousStateAttributes=''  FilterStateMustResolveToSignalObject=off  FilterRTWStateStorageClass=Auto  ParallelPVariant=ExternalParameters  IdealPVariant=Disabled  IVariant=ExternalParameters  DVariant=Disabled  IntegratorVariant=Discrete  SatVariant=Enabled  AWVariant=DiscClampingParallel  PCopyVariant=Disabled  TRVariant=Disabled  FdbkBlocksVariant=Forward  IdealPFdbkVariant=Disabled  SatFdbkVariant=Disabled  DerivativeFilterVariant=Disabled  NVariant=Disabled  NCopyVariant=Disabled_SignalSpec  FilterICVariant=Disabled  IntegratorICVariant=InternalICs  ExternalResetVariant=Disabled  TRSumVariant=Passthrough  SumFdbkVariant=Disabled  SumVariant=Sum_PI  TsampFilterVariant=InternalTs  TsampNgainVariant=Passthrough  TsampIntegralVariant=Disabled_SignalSpec  ExternalSaturationOutDataTypeStr=Inherit: Same as second input  DerivativeSourceVariant=Disabled
      settings: LibrarySourceBlock=simulink/Discrete/Discrete PID Controller
  Sum : Sum  Inputs=+-|
  SpeedPID_Out : Outport
  wires:
  Sum/1 -> Discrete PID Controller/1
  Speed_Kp/1 -> Discrete PID Controller/2
  Speed_Ref/1 -> Sum/1
  Discrete PID Controller/1 -> SpeedPID_Out/1
  Speed_Ki/1 -> Discrete PID Controller/3
  Speed_Real/1 -> Sum/2

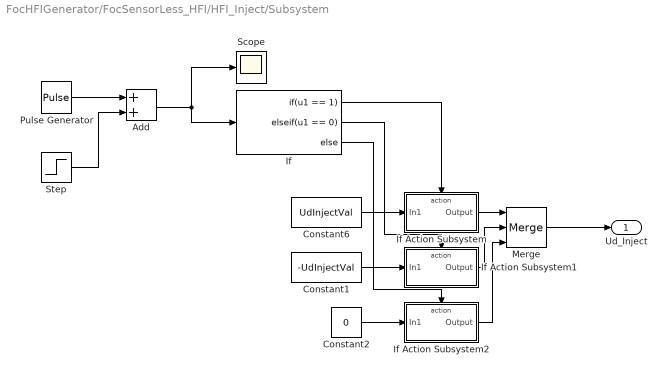
== system FocHFIGenerator/FocSensorLess_HFI/HFI_Inject/Subsystem ==
  Add : Sum
  Constant1 : Constant  Value=-UdInjectVal  OutDataTypeStr=single
  Constant2 : Constant  Value=0  OutDataTypeStr=single
  Constant6 : Constant  Value=UdInjectVal  OutDataTypeStr=single
  If : If  IfExpression=u1 == 1  ElseIfExpressions=u1 == 0
  If Action Subsystem : Subsystem  TreatAsAtomicUnit=on
  If Action Subsystem1 : Subsystem  TreatAsAtomicUnit=on
  If Action Subsystem2 : Subsystem  TreatAsAtomicUnit=on
  Merge : Merge  Inputs=3
  Pulse Generator : DiscretePulseGenerator  PulseType=Time based  Period=0.0001  PulseWidth=50  PhaseDelay=0.2
  Scope : Scope
  Step : Step  Time=0.2  Before=5  After=0  SampleTime=0
  Ud_Inject : Outport
  wires:
  Merge/1 -> Ud_Inject/1
  Constant1/1 -> If Action Subsystem1/1(In1)
  If Action Subsystem/1(Output) -> Merge/1
  If Action Subsystem1/1(Output) -> Merge/2
  Constant6/1 -> If Action Subsystem/1(In1)
  Pulse Generator/1 -> Add/1
  Add/1 -> Scope/1, If/1
  Step/1 -> Add/2
  If/1 -> If Action Subsystem/Action
  If/2 -> If Action Subsystem1/Action
  If/3 -> If Action Subsystem2/Action
  If Action Subsystem2/1(Output) -> Merge/3
  Constant2/1 -> If Action Subsystem2/1(In1)

== system FocHFIGenerator/FocSensorLess_HFI/HFI_Inject/Subsystem4 ==
  Add1 : Sum  Inputs=+-  OutDataTypeStr=single  AccumDataTypeStr=single
  Add2 : Sum  Inputs=+-  OutDataTypeStr=single  AccumDataTypeStr=single
  Scope : Scope
  Scope1 : Scope
  Scope2 : Scope
  Step1 : Step  Time=0.13  After=-2  OutDataTypeStr=single  SampleTime=0
  Step2 : Step  Time=0.14  After=-2  OutDataTypeStr=single  SampleTime=0
  Step3 : Step  Time=0.1  After=2  OutDataTypeStr=single  SampleTime=0
  Step4 : Step  Time=0.11  After=2  OutDataTypeStr=single  SampleTime=0
  Sum : Sum  Inputs=+|+
  NDS_Signal : Outport
  wires:
  Add2/1 -> Sum/2, Scope1/1
  Step1/1 -> Add2/1
  Step2/1 -> Add2/2
  Step3/1 -> Add1/1
  Add1/1 -> Sum/1, Scope/1
  Step4/1 -> Add1/2
  Sum/1 -> Scope2/1, NDS_Signal/1

== system FocHFIGenerator/FocSensorLess_HFI/NSD/Subsystem ==
  Input : Inport
  Trigger : TriggerPort  VariantControl=(inherit)  PortDimensions=1
  Output : Outport
  wires:
  Input/1 -> Output/1

== system FocHFIGenerator/FocSensorLess_HFI/SVPWM/InvClark ==
  Ualpha : Inport  OutDataTypeStr=single
  Ubeta : Inport  Port=2  OutDataTypeStr=single
  Gain : Gain  Gain=-1/2  OutDataTypeStr=single
  Gain1 : Gain  Gain=sqrt(3)/2  OutDataTypeStr=single
  Sum : Sum  Inputs=|++  OutDataTypeStr=single
  Sum1 : Sum  Inputs=-+|  OutDataTypeStr=single
  Ua : Outport  OutDataTypeStr=single
  Ub : Outport  Port=2  OutDataTypeStr=single
  Uc : Outport  Port=3  OutDataTypeStr=single
  wires:
  Ualpha/1 -> Gain/1, Ua/1
  Ubeta/1 -> Gain1/1
  Gain/1 -> Sum1/2, Sum/1
  Sum/1 -> Ub/1
  Gain1/1 -> Sum/2, Sum1/1
  Sum1/1 -> Uc/1

== system FocHFIGenerator/FocSensorLess_HFI/SVPWM/ei_t ==
  Uabc : Inport  OutDataTypeStr=single
  Demux : Demux  Outputs=3
  Gain : Gain  Gain=-1/2  OutDataTypeStr=single
  Min : MinMax  Inputs=3  OutDataTypeStr=single
  Min1 : MinMax  Function=max  Inputs=3  OutDataTypeStr=single
  Sum : Sum  Inputs=|++  OutDataTypeStr=single
  ei_t : Outport  OutDataTypeStr=single
  wires:
  Min/1 -> Sum/1
  Sum/1 -> Gain/1
  Min1/1 -> Sum/2
  Gain/1 -> ei_t/1
  Uabc/1 -> Demux/1
  Demux/1 -> Min1/1, Min/1
  Demux/2 -> Min/2, Min1/2
  Demux/3 -> Min1/3, Min/3

== system FocHFIGenerator/FocSensorLess_HFI/HFI_Inject/Subsystem/If Action Subsystem ==
  In1 : Inport
  Action Port : ActionPort  ActionPortLabel=if(u1 == 1)
  Output : Outport
  wires:
  In1/1 -> Output/1

== system FocHFIGenerator/FocSensorLess_HFI/HFI_Inject/Subsystem/If Action Subsystem1 ==
  In1 : Inport
  Action Port : ActionPort  ActionPortLabel=elseif(u1 == 0)
  Output : Outport
  wires:
  In1/1 -> Output/1

== system FocHFIGenerator/FocSensorLess_HFI/HFI_Inject/Subsystem/If Action Subsystem2 ==
  In1 : Inport
  Action Port : ActionPort  ActionPortLabel=else
  Output : Outport
  wires:
  In1/1 -> Output/1
